simulink model "MCR2_Example_Publisher_Subscriber"  (R2024a)
settings: Solver=VariableStepAuto  StartTime=0.0  StopTime=Inf  RelTol=1e-3
libraries: robotlib x3
settings Model: Creator=mario  LastModifiedBy=mario

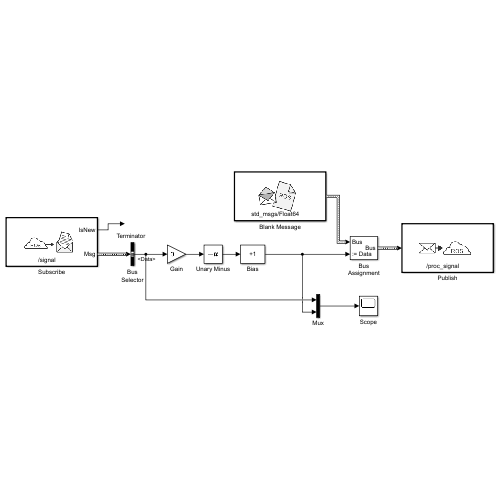
[thumbnail: Simulink's stored preview of the top-level diagram]
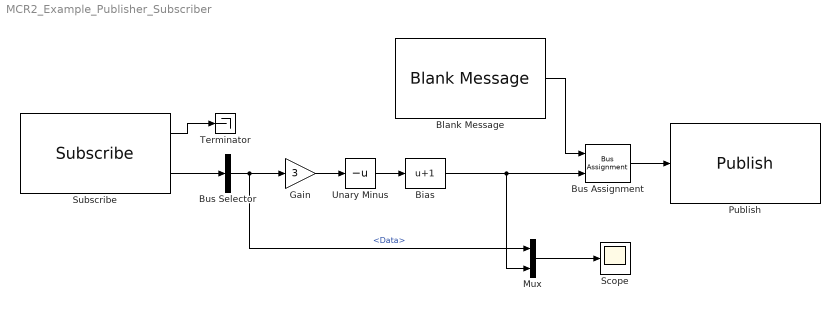
== system MCR2_Example_Publisher_Subscriber ==
  Bias : Bias  Bias=1  SaturateOnIntegerOverflow=off
  Blank Message : robotlib/Blank Message  messageClass=Message  entityType=std_msgs/Float64  messageType=std_msgs/Float64  SampleTime=0.01  legacyBusStruct=off
  Bus Assignment : BusAssignment  AssignedSignals=Data
  Bus Selector : BusSelector  OutputSignals=Data
  Gain : Gain  Gain=3
  Mux : Mux  Inputs=2
  Publish : robotlib/Publish  topicSource=Specify your own  topic=/proc_signal  messageType=std_msgs/Float64  legacyBusStruct=off  messageQueueLength=1
  Scope : Scope
  Subscribe : robotlib/Subscribe  topicSource=Specify your own  topic=/signal  messageType=std_msgs/Float64  SampleTime=0.01  legacyBusStruct=off  messageQueueLength=1
  Terminator : Terminator
  Unary Minus : UnaryMinus
  wires:
  Subscribe/2 -> Bus Selector/1
  Subscribe/1 -> Terminator/1
  Bus Selector/1 -> Mux/1, Gain/1  "<Data>"
  Bus Assignment/1 -> Publish/1
  Blank Message/1 -> Bus Assignment/1
  Unary Minus/1 -> Bias/1
  Gain/1 -> Unary Minus/1
  Bias/1 -> Bus Assignment/2, Mux/2
  Mux/1 -> Scope/1
